simulink model "Synch_Gen"  (Simulink 4.00)
settings: Solver=ode23tb  StartTime=0.0  StopTime=1
InitFcn:
  | powericon('psbinitsys',bdroot);
libraries: powerlib2 x4, powerlib_extras x3
settings Model: SaveTime=off  SaveOutput=off  LimitDataPoints=off  BlockReductionOpt=off

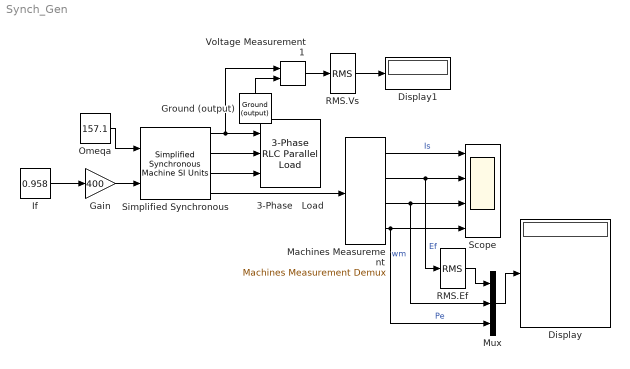
== system Synch_Gen ==
  3-Phase   Load : powerlib_extras/Three-Phase Library/3-Phase RLC Parallel Load  Vpp=380  fn=50  P3=100e3*0.1  QL3=0  QC3=100e3*0.1
  Display : Display
      settings: Format=short  SampleTime=0
  Display1 : Display
      settings: Format=short  SampleTime=0
  Gain : Gain  Gain=400  Multiplication=Element-wise(K.*u)  SaturateOnIntegerOverflow=on
  Ground (output) : powerlib2/Connectors/Ground (output)  Tag=PoWeRsYsTeMbLoCk  Orientation=up  PSBOutputType=1
  If : Constant  Value=0.958
  Machines Measurement : powerlib2/Machines/Machines Measurement Demux  machType=Simplified synchronous  ssm1=on  ssm2=off  ssm3=on  ssm4=off  ssm5=on  ssm6=on  sm1=on  sm2=off  sm3=on  sm4=off  sm5=off  sm6=off  sm7=off  sm8=on  sm9=on  sm10=off  sm11=off  asm1=on  asm2=on  asm3=on  asm4=on  asm5=on  asm6=on  asm7=on  asm8=on  asm9=on  asm10=on  asm11=on  pmsm1=on  pmsm2=on  pmsm3=on  pmsm4=on  pmsm5=on  pmsm6=on  lastType=1
  Mux : Mux  Inputs=3
  Omeqa : Constant  Value=157.1
  RMS.Ef : powerlib_extras/Measurements/RMS  f1=50
  RMS.Vs : powerlib_extras/Measurements/RMS  f1=50
  Scope : Scope  NumInputPorts=4
      settings: TimeRange=auto  YMin=-400~-400~268.606~0  YMax=400~400~296.88~150000  SaveToWorkspace=off  SaveName=ScopeData  MaxDataPoints=5000
  "Simplified Synchronous " : powerlib2/Machines/Simplified Synchronous  Machine SI Units  Tag=PoWeRsYsTeMbLoCk  conType=3-wire Y  x1=[ 100e3,380,50 ]  x2=[ inf,0,2 ]  x3=[ 0. 0.9e-3 ]  x4="[ 0   0   0,0,0   0,0,0 ]"  PSBOutputType=1111  iounits=1
  Voltage Measurement1 : powerlib2/Measurements/Voltage Measurement  Tag=PoWeRsYsTeMmEaSuReMeNt  PSBOutputType=0  PSBequivalent=1
  wires:
  "Simplified Synchronous "/1 -> 3-Phase   Load/1, Voltage Measurement1/1
  "Simplified Synchronous "/2 -> 3-Phase   Load/2
  "Simplified Synchronous "/3 -> 3-Phase   Load/3
  "Simplified Synchronous "/4 -> Machines Measurement/1
  Omeqa/1 -> "Simplified Synchronous "/1
  Machines Measurement/1 -> Scope/1  "Is"
  Voltage Measurement1/1 -> RMS.Vs/1
  RMS.Vs/1 -> Display1/1
  Ground (output)/1 -> Voltage Measurement1/2
  Machines Measurement/2 -> Scope/2, RMS.Ef/1  "Ef"
  Machines Measurement/3 -> Scope/3, Mux/2  "wm"
  Machines Measurement/4 -> Scope/4, Mux/3  "Pe"
  RMS.Ef/1 -> Mux/1
  Mux/1 -> Display/1
  If/1 -> Gain/1
  Gain/1 -> "Simplified Synchronous "/2
